simulink model "s0208"  (Simulink 6.0)
settings: Solver=ode45  SolverMode=SingleTasking  StartTime=0.0  StopTime=5  MaxStep=.1  RelTol=1e-3  AbsTol=1e-6
values from neighbouring files (symbols this model uses):
  Aab0 = Aab0*1e-6    (= 6e-06)    [m0208.m]    (also in m0221d.m; m0224.m)
  uPdach = uP(i)    [m0208.m]
settings Model: LastModifiedBy=Froriep
settings DataIOCC: LimitDataPoints=off  SaveOutput=off  TimeSaveName=t  SignalLoggingName=sigsOut
settings OptimizationCC: BooleanDataType=off
settings DebuggingCC: SolverPrmCheckMsg=none
settings HardwareCC: TargetUnknown=on
settings GRTTargetCC: ModelReferenceCompliant=off  MatFileLogging=off

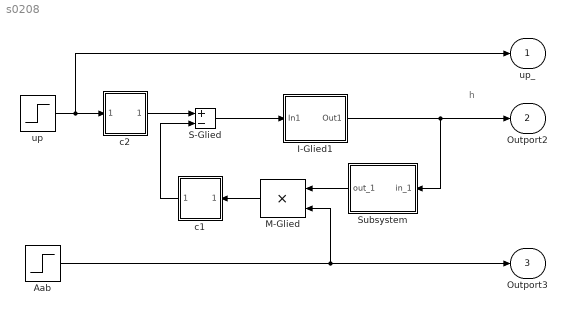
== system s0208 ==
  note: h
  Aab : Step  Time=0  Before=Aab0  After=Aab0  SampleTime=0
  I-Glied1 : Subsystem  mask(I-Glied){@1=0}
      mask prompts: @1 "Anfangswert"
      mask help: I-Glied
      mask init:
      | x0=@1;
      mask Display: disp('I-Glied')
  M-Glied : Product  Orientation=left  SaturateOnIntegerOverflow=on  RndMeth=Zero  InputSameDT=on
  S-Glied : Sum  Inputs=+-  SaturateOnIntegerOverflow=on  InputSameDT=on
  Subsystem : Subsystem  Orientation=left
      mask Display: disp('Wurzel')
  c1 : Subsystem  Orientation=left  mask(P-Glied){@1=c1}
      mask prompts: @1 "Beiwert"
      mask help: P-Glied
      mask init:
      | Kp=@1;
      mask Display: disp('c1')
  c2 : Subsystem  mask(P-Glied){@1=c2}
      mask prompts: @1 "Beiwert"
      mask help: P-Glied
      mask init:
      | Kp=@1;
      mask Display: disp('c2')
  up : Step  Time=50  After=uPdach  SampleTime=0
  up_ : Outport
  Outport2 : Outport  Port=2
  Outport3 : Outport  Port=3
  wires:
  c2/1(Out1) -> S-Glied/1
  S-Glied/1 -> I-Glied1/1(In1)
  M-Glied/1 -> c1/1(In1)
  Subsystem/1(out_1) -> M-Glied/1
  c1/1(Out1) -> S-Glied/2
  up/1 -> up_/1, c2/1(In1)
  I-Glied1/1(Out1) -> Outport2/1, Subsystem/1(in_1)
  Aab/1 -> M-Glied/2, Outport3/1

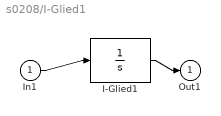
== system s0208/I-Glied1 ==
  In1 : Inport  Port=1  LatchInput=off
  I-Glied1 : Integrator  InitialCondition=x0
  Out1 : Outport
  wires:
  I-Glied1/1 -> Out1/1
  In1/1 -> I-Glied1/1

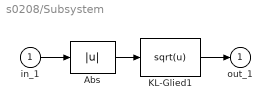
== system s0208/Subsystem ==
  in_1 : Inport  Port=1  LatchInput=off
  Abs : Abs  SaturateOnIntegerOverflow=on
  KL-Glied1 : Fcn  Expr=sqrt(u)
  out_1 : Outport
  wires:
  KL-Glied1/1 -> out_1/1
  in_1/1 -> Abs/1
  Abs/1 -> KL-Glied1/1

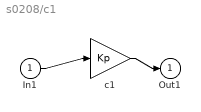
== system s0208/c1 ==
  In1 : Inport  Port=1  LatchInput=off
  c1 : Gain  Gain=Kp  SaturateOnIntegerOverflow=on
  Out1 : Outport
  wires:
  c1/1 -> Out1/1
  In1/1 -> c1/1

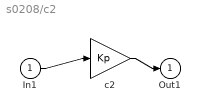
== system s0208/c2 ==
  In1 : Inport  Port=1  LatchInput=off
  c2 : Gain  Gain=Kp  SaturateOnIntegerOverflow=on
  Out1 : Outport
  wires:
  c2/1 -> Out1/1
  In1/1 -> c2/1
